simulink model "prob_9"  (R2015a)
settings: Solver=ode45  StartTime=0.0  StopTime=2  RelTol=1e-3
libraries: simulink x1
settings Model: Creator=Anu  LastModifiedBy=Anu

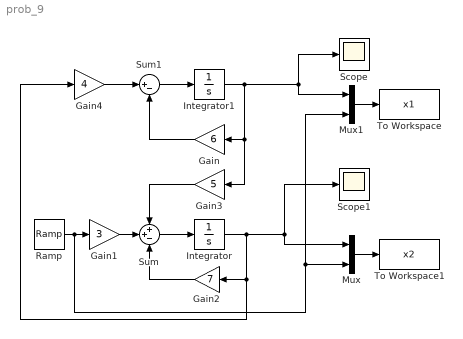
== system prob_9 ==
  Gain : Gain  Gain=6
  Gain1 : Gain  Gain=3
  Gain2 : Gain  Gain=7
  Gain3 : Gain  Gain=5
  Gain4 : Gain  Gain=4
  Integrator : Integrator
  Integrator1 : Integrator
  Mux : Mux  Inputs=2
  Mux1 : Mux  Inputs=2
  Ramp : simulink/Sources/Ramp  slope=1  start=0  X0=0
  Scope : Scope
  Scope1 : Scope
  Sum : Sum  Inputs=++-
  Sum1 : Sum  Inputs=|+-
  To Workspace : ToWorkspace  VariableName=x1  SampleTime=-1
  To Workspace1 : ToWorkspace  VariableName=x2  SampleTime=-1
  wires:
  Gain4/1 -> Sum1/1
  Sum1/1 -> Integrator1/1
  Integrator1/1 -> Mux1/1, Scope/1, Gain3/1, Gain/1
  Gain/1 -> Sum1/2
  Gain3/1 -> Sum/1
  Gain1/1 -> Sum/2
  Ramp/1 -> Mux/2, Mux1/2, Gain1/1
  Sum/1 -> Integrator/1
  Integrator/1 -> Gain4/1, Gain2/1, Mux/1, Scope1/1
  Gain2/1 -> Sum/3
  Mux/1 -> To Workspace1/1
  Mux1/1 -> To Workspace/1
